simulink model "Rail_PreCtlMeUn"  (R2016b)
settings: configuration reference "CodeGenConfigSet" (kept outside this file)
values from neighbouring files (symbols this model uses):
  Epm_numCyl_C = Calibration.Parameter    [init_Rail_PreCtlMeUn.m]    (also in init_Rail_PreCtlMeUn_SIL.m = Simulink.Parameter)
  PCV_dvolLeak_C = Calibration.Parameter    [init_Rail_PreCtlMeUn.m]    (also in init_Rail_PreCtlMeUn_SIL.m = Simulink.Parameter)
  Rail_dvolLeak_CUR = Calibration.Parameter    [init_Rail_PreCtlMeUn.m]    (also in init_Rail_PreCtlMeUn_SIL.m = Simulink.Parameter)
  Rail_dvolLeak_CURX = Calibration.Parameter    [init_Rail_PreCtlMeUn.m]    (also in init_Rail_PreCtlMeUn_SIL.m = Simulink.Parameter)
  Rail_facDemInjCtlMax_C = Calibration.Parameter    [init_Rail_PreCtlMeUn.m]    (also in init_Rail_PreCtlMeUn_SIL.m = Simulink.Parameter)
  Rail_facLeakEngOn_CUR = Calibration.Parameter    [init_Rail_PreCtlMeUn.m]    (also in init_Rail_PreCtlMeUn_SIL.m = Simulink.Parameter)
  Rail_facLeakEngOn_CURX = Calibration.Parameter    [init_Rail_PreCtlMeUn.m]    (also in init_Rail_PreCtlMeUn_SIL.m = Simulink.Parameter)
  Rail_facLeakTempCor_CUR = Calibration.Parameter    [init_Rail_PreCtlMeUn.m]    (also in init_Rail_PreCtlMeUn_SIL.m = Simulink.Parameter)
  Rail_facLeakTempCor_CURX = Calibration.Parameter    [init_Rail_PreCtlMeUn.m]    (also in init_Rail_PreCtlMeUn_SIL.m = Simulink.Parameter)
  Rail_facPreCtlMeUnCor_MAP = Calibration.Parameter    [init_Rail_PreCtlMeUn.m]    (also in init_Rail_PreCtlMeUn_SIL.m = Simulink.Parameter)
  Rail_facPreCtlMeUnCor_MAPX = Calibration.Parameter    [init_Rail_PreCtlMeUn.m]    (also in init_Rail_PreCtlMeUn_SIL.m = Simulink.Parameter)
  Rail_facPreCtlMeUnCor_MAPY = Calibration.Parameter    [init_Rail_PreCtlMeUn.m]    (also in init_Rail_PreCtlMeUn_SIL.m = Simulink.Parameter)
  Rail_numInjSum_C = Calibration.Parameter    [init_Rail_PreCtlMeUn.m]    (also in init_Rail_PreCtlMeUn_SIL.m = Simulink.Parameter)
  Rail_PreCtlDynKd_C = Calibration.Parameter    [init_Rail_PreCtlMeUn.m]    (also in init_Rail_PreCtlMeUn_SIL.m = Simulink.Parameter)
  Rail_qDemInjCtl_CUR = Calibration.Parameter    [init_Rail_PreCtlMeUn.m]    (also in init_Rail_PreCtlMeUn_SIL.m = Simulink.Parameter)
  Rail_qDemInjCtl_CURX = Calibration.Parameter    [init_Rail_PreCtlMeUn.m]    (also in init_Rail_PreCtlMeUn_SIL.m = Simulink.Parameter)
  Rail_qDemInjCtlMaxOfs_C = Calibration.Parameter    [init_Rail_PreCtlMeUn.m]    (also in init_Rail_PreCtlMeUn_SIL.m = Simulink.Parameter)
  Rail_qPreCtlDynDiffMin_C = Calibration.Parameter    [init_Rail_PreCtlMeUn.m]    (also in init_Rail_PreCtlMeUn_SIL.m = Simulink.Parameter)
  Rail_swtDemInjSel_C = Calibration.Parameter    [init_Rail_PreCtlMeUn.m]    (also in init_Rail_PreCtlMeUn_SIL.m = Simulink.Parameter)
  Rail_tiPreCtlDynT1_C = Calibration.Parameter    [init_Rail_PreCtlMeUn.m]    (also in init_Rail_PreCtlMeUn_SIL.m = Simulink.Parameter)
undefined symbols (not defined in the file or in its folder): EngState_conv, EpmSynState_conv, Rail_PreCtlMeUn_DT
libraries: CXLib x2
settings Model: Creator=lenovo  LastModifiedBy=mayongchao
settings ConfigSetRef: SourceLocation=Base Workspace

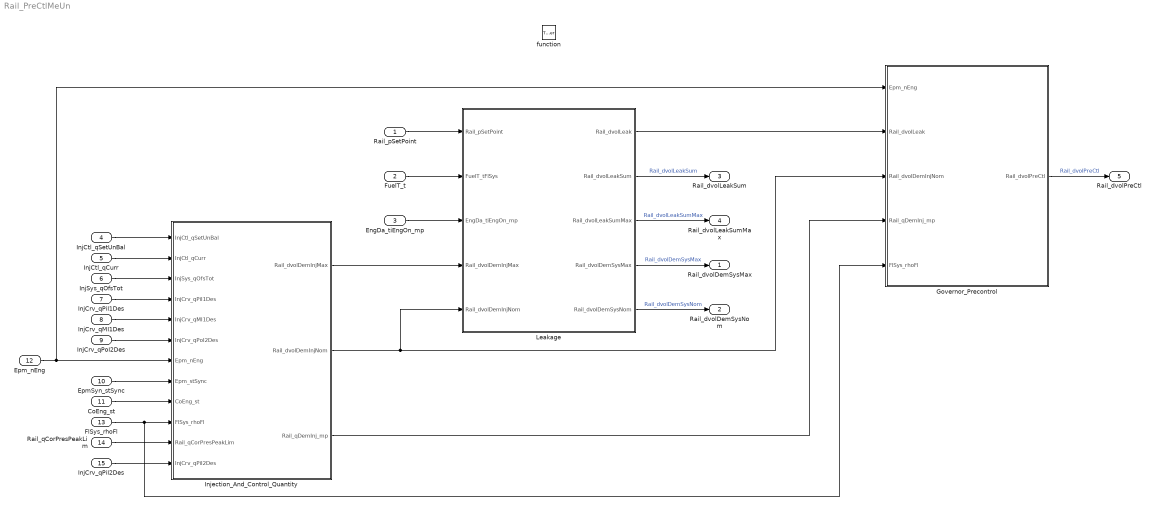
== system Rail_PreCtlMeUn ==
  Rail_pSetPoint : Inport  Tag=bar  Description=Rail pressure setpoint  OutMin=-2500  OutMax=2500  OutDataTypeStr=RailPressure_bar
  FuelT_t : Inport  Tag=deg  Description=Temperature of fuel  Port=2  OutMin=-50  OutMax=150  OutDataTypeStr=Temp_deg
  EngDa_tiEngOn_mp : Inport  Tag=s  Description=Engine on time  Port=3  OutMin=-2147483648  OutMax=2147483647  OutDataTypeStr=TimeEngOn_s
  InjCtl_qSetUnBal : Inport  Tag=mg/hub  Description=Current injection quantity  Port=4  OutMin=-319  OutMax=319  OutDataTypeStr=FuelMass_mg_hub
  InjCtl_qCurr : Inport  Tag=mg/hub  Description=Torque generating engine fuel injection quantity  Port=5  OutMin=-319  OutMax=319  OutDataTypeStr=FuelMass_mg_hub
  InjSys_qOfsTot : Inport  Tag=mg/hub  Description=Non-torque generating quantity, the offset-quantity from torque generating quantity to total quantity  Port=6  OutMin=-319  OutMax=319  OutDataTypeStr=FuelMass_mg_hub
  InjCrv_qPiI1Des : Inport  Tag=mg/hub  Description=Desired PiI injection quantity  Port=7  OutMin=-319  OutMax=319  OutDataTypeStr=FuelMass_mg_hub
  InjCrv_qMI1Des : Inport  Tag=mg/hub  Description=desired MI1 injection quantity  Port=8  OutMin=-319  OutMax=319  OutDataTypeStr=FuelMass_mg_hub
  InjCrv_qPoI2Des : Inport  Tag=mg/hub  Description=Desired PoI2 injection quantity  Port=9  OutMin=-319  OutMax=319  OutDataTypeStr=FuelMass_mg_hub
  EpmSyn_stSync : Inport  Description=state of synchronization  Port=10  OutDataTypeStr=Enum: EpmSynState_conv
  CoEng_st : Inport  Description=Engine coordinator state  Port=11  OutDataTypeStr=Enum: EngState_conv
  Epm_nEng : Inport  Tag=rpm  Description=Engine speed  Port=12  OutMin=0  OutMax=6000  OutDataTypeStr=EngSpeed_rpm
  FlSys_rhoFl : Inport  Tag=kg/m^3  Description=Fuel density coefficient  Port=13  OutMin=0  OutMax=3276  OutDataTypeStr=Fuel_Rho_kg_m3
  Rail_qCorPresPeakLim : Inport  Tag=mg/hub  Description=Quantity correction for limiting pressure peaks (pos. and neg.) mg/cyc  RequirementInfo={'other' 'Rail_requirements.doc' '@Simulink_requirement_item_21' 'true' '（1）根据需求油量选择开关Rail_swtDemInjSel_C选择相应的喷油量作为需求油量。' '' } %GIDa_61847e45_e1c1_4d7b_9351_12b0d31b0ef4  Port=14  OutMin=-300  OutMax=300  OutDataTypeStr=FuelMass_mg_hub
  InjCrv_qPiI2Des : Inport  Tag=mg/hub  Description=Desired PiI injection quantity  RequirementInfo={'other' 'Rail_requirements.doc' '@Simulink_requirement_item_22' 'true' '（2）根据预喷油量和主喷油量查表Rail_qDemInjCtl_CUR，得到相应的控制油量，将两个控制油量相加得到总的控制油量Rail_qDemInjCtlNom_mp。' '' } %GIDa_2488a317_7988_4bfa_9d08_9b42b553773c  Port=15  OutMin=-319  OutMax=319  OutDataTypeStr=FuelMass_mg_hub
  function : TriggerPort  TriggerType=function-call  VariantControl=Variant
  Governor_Precontrol : Subsystem
  Injection_And_Control_Quantity : Subsystem
  Leakage : Subsystem
  Rail_dvolDemSysMax : Outport  Tag=mm^3/s  Description=Volume flow requested overall for a maximum tolerated injection system  OutMin=-327680  OutMax=327670  OutDataTypeStr=FuelVol_mm3_s
  Rail_dvolDemSysNom : Outport  Tag=mm^3/s  Description=Volume flow demanded overall for a nominal injection system  Port=2  OutMin=-327680  OutMax=327670  OutDataTypeStr=FuelVol_mm3_s
  Rail_dvolLeakSum : Outport  Tag=mm^3/s  Description=Summary of Leakages  Port=3  OutMin=-327680  OutMax=327670  OutDataTypeStr=FuelVol_mm3_s
  Rail_dvolLeakSumMax : Outport  Tag=mm^3/s  Description=Lifetime dependant maximum estimated system leakage  Port=4  OutMin=-327680  OutMax=327670  OutDataTypeStr=FuelVol_mm3_s
  Rail_dvolPreCtl : Outport  Tag=mm^3/s  Description=Precontrol value for pressure governing by metering unit  Port=5  OutMin=-327680  OutMax=327670  OutDataTypeStr=FuelVol_mm3_s
  wires:
  Injection_And_Control_Quantity/3(Rail_qDemInj_mp) -> Governor_Precontrol/4(Rail_qDemInj_mp)
  FlSys_rhoFl/1 -> Governor_Precontrol/5(FlSys_rhoFl), Injection_And_Control_Quantity/10(FlSys_rhoFl)
  Governor_Precontrol/1(Rail_dvolPreCtl) -> Rail_dvolPreCtl/1  "Rail_dvolPreCtl"
  Injection_And_Control_Quantity/2(Rail_dvolDemInjNom) -> Leakage/5(Rail_dvolDemInjNom), Governor_Precontrol/3(Rail_dvolDemInjNom)
  Leakage/5(Rail_dvolDemSysNom) -> Rail_dvolDemSysNom/1  "Rail_dvolDemSysNom"
  Leakage/4(Rail_dvolDemSysMax) -> Rail_dvolDemSysMax/1  "Rail_dvolDemSysMax"
  Leakage/3(Rail_dvolLeakSumMax) -> Rail_dvolLeakSumMax/1  "Rail_dvolLeakSumMax"
  Leakage/2(Rail_dvolLeakSum) -> Rail_dvolLeakSum/1  "Rail_dvolLeakSum"
  Leakage/1(Rail_dvolLeak) -> Governor_Precontrol/2(Rail_dvolLeak)
  CoEng_st/1 -> Injection_And_Control_Quantity/9(CoEng_st)
  EpmSyn_stSync/1 -> Injection_And_Control_Quantity/8(Epm_stSync)
  Epm_nEng/1 -> Governor_Precontrol/1(Epm_nEng), Injection_And_Control_Quantity/7(Epm_nEng)
  InjCrv_qMI1Des/1 -> Injection_And_Control_Quantity/5(InjCrv_qMI1Des)
  InjCrv_qPiI1Des/1 -> Injection_And_Control_Quantity/4(InjCrv_qPiI1Des)
  InjSys_qOfsTot/1 -> Injection_And_Control_Quantity/3(InjSys_qOfsTot)
  InjCtl_qSetUnBal/1 -> Injection_And_Control_Quantity/1(InjCtl_qSetUnBal)
  InjCtl_qCurr/1 -> Injection_And_Control_Quantity/2(InjCtl_qCurr)
  FuelT_t/1 -> Leakage/2(FuelT_tFlSys)
  EngDa_tiEngOn_mp/1 -> Leakage/3(EngDa_tiEngOn_mp)
  Rail_pSetPoint/1 -> Leakage/1(Rail_pSetPoint)
  Injection_And_Control_Quantity/1(Rail_dvolDemInjMax) -> Leakage/4(Rail_dvolDemInjMax)
  InjCrv_qPoI2Des/1 -> Injection_And_Control_Quantity/6(InjCrv_qPoI2Des)
  Rail_qCorPresPeakLim/1 -> Injection_And_Control_Quantity/11(Rail_qCorPresPeakLim)
  InjCrv_qPiI2Des/1 -> Injection_And_Control_Quantity/12(InjCrv_qPiI2Des)

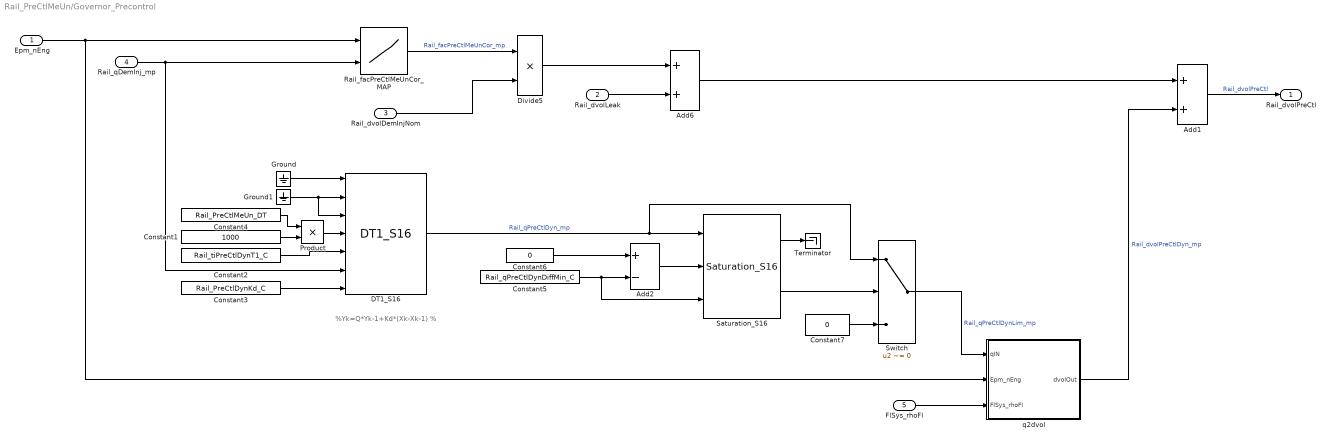
== system Rail_PreCtlMeUn/Governor_Precontrol ==
  note: %Yk=Q*Yk-1+Kd*(Xk-Xk-1) %
  Epm_nEng : Inport  RequirementInfo={'other' 'Rail_requirements.doc' '@Simulink_requirement_item_33' 'true' '基础前馈值' '' } %GIDa_7183900f_2547_4057_a7ba_251e952e1021
  Rail_dvolLeak : Inport  RequirementInfo={'other' 'Rail_requirements.doc' '@Simulink_requirement_item_33' 'true' '基础前馈值' '' } %GIDa_3503d7f1_41ae_4a42_98db_e3eecb9170cb  Port=2
  Rail_dvolDemInjNom : Inport  RequirementInfo={'other' 'Rail_requirements.doc' '@Simulink_requirement_item_33' 'true' '基础前馈值' '' } %GIDa_868a355a_ff47_4d62_936b_22abb35e9b86  Port=3
  Rail_qDemInj_mp : Inport  RequirementInfo={'other' 'Rail_requirements.doc' '@Simulink_requirement_item_33' 'true' '基础前馈值' '' } %GIDa_e1428e79_ed0e_4ba1_a3fd_0a41696d3c11  Port=4
  FlSys_rhoFl : Inport  RequirementInfo={'other' 'Rail_requirements.doc' '@Simulink_requirement_item_34' 'true' '前馈动态补偿体积Rail_dvolPreCtlDyn_mp' '' } %GIDa_798c307b_f932_4494_bf5f_3947ced32dad  Port=5
  Add1 : Sum  InputSameDT=on
  Add2 : Sum  RequirementInfo={'other' 'Rail_requirements.doc' '@Simulink_requirement_item_34' 'true' '前馈动态补偿体积Rail_dvolPreCtlDyn_mp' '' } %GIDa_11a574b0_8317_4258_b280_8d8a7cfa794e  Inputs=+-  InputSameDT=on
  Add6 : Sum  RequirementInfo={'other' 'Rail_requirements.doc' '@Simulink_requirement_item_33' 'true' '基础前馈值' '' } %GIDa_f82aefef_e4ab_49af_af00_2d184f409336  InputSameDT=on
  Constant1 : Constant  RequirementInfo={'other' 'Rail_requirements.doc' '@Simulink_requirement_item_34' 'true' '前馈动态补偿体积Rail_dvolPreCtlDyn_mp' '' } %GIDa_e791a252_ee7e_42c9_85f3_a169ed1ddcc4  Value=1000  OutDataTypeStr=uint16
  Constant2 : Constant  RequirementInfo={'other' 'Rail_requirements.doc' '@Simulink_requirement_item_34' 'true' '前馈动态补偿体积Rail_dvolPreCtlDyn_mp' '' } %GIDa_ec4b6c88_d6b6_478e_9290_0243aa0efb63  Value=Rail_tiPreCtlDynT1_C
  Constant3 : Constant  RequirementInfo={'other' 'Rail_requirements.doc' '@Simulink_requirement_item_34' 'true' '前馈动态补偿体积Rail_dvolPreCtlDyn_mp' '' } %GIDa_c4a7ef06_b727_4a3d_94c2_08782c9b8867  Value=Rail_PreCtlDynKd_C
  Constant4 : Constant  RequirementInfo={'other' 'Rail_requirements.doc' '@Simulink_requirement_item_34' 'true' '前馈动态补偿体积Rail_dvolPreCtlDyn_mp' '' } %GIDa_1b5483ab_5d1d_41df_9217_4aee7852aaf8  Value=Rail_PreCtlMeUn_DT  OutDataTypeStr=uint16
  Constant5 : Constant  RequirementInfo={'other' 'Rail_requirements.doc' '@Simulink_requirement_item_34' 'true' '前馈动态补偿体积Rail_dvolPreCtlDyn_mp' '' } %GIDa_54dd0a63_7d23_407e_aac7_70a39433bdd0  Value=Rail_qPreCtlDynDiffMin_C
  Constant6 : Constant  RequirementInfo={'other' 'Rail_requirements.doc' '@Simulink_requirement_item_34' 'true' '前馈动态补偿体积Rail_dvolPreCtlDyn_mp' '' } %GIDa_20ac7aa5_ee3b_45c0_9ed5_4f6856be27d3  Value=0  OutDataTypeStr=Inherit: Inherit via back propagation
  Constant7 : Constant  RequirementInfo={'other' 'Rail_requirements.doc' '@Simulink_requirement_item_34' 'true' '前馈动态补偿体积Rail_dvolPreCtlDyn_mp' '' } %GIDa_dbe14c56_3d27_499d_a0c9_6c8275566cb4  Value=0  OutDataTypeStr=Inherit: Inherit via back propagation
  DT1_S16 : CXLib/DT1_S16  RequirementInfo={'other' 'Rail_requirements.doc' '@Simulink_requirement_item_34' 'true' '前馈动态补偿体积Rail_dvolPreCtlDyn_mp' '' } %GIDa_61af2057_1ae7_4294_9d8b_88d75294bae1
  Divide5 : Product  RequirementInfo={'other' 'Rail_requirements.doc' '@Simulink_requirement_item_33' 'true' '基础前馈值' '' } %GIDa_4ce6a312_6fe6_46db_860a_63764939d657  Inputs=**  OutDataTypeStr=FuelVol_mm3_s
  Ground : Ground  RequirementInfo={'other' 'Rail_requirements.doc' '@Simulink_requirement_item_34' 'true' '前馈动态补偿体积Rail_dvolPreCtlDyn_mp' '' } %GIDa_0a4a3791_a005_4ed8_981b_586e8985940b
  Ground1 : Ground  RequirementInfo={'other' 'Rail_requirements.doc' '@Simulink_requirement_item_34' 'true' '前馈动态补偿体积Rail_dvolPreCtlDyn_mp' '' } %GIDa_2de3f24a_c7b3_45e3_9504_81736252fde4
  Product : Product  OutDataTypeStr=uint32
  Rail_facPreCtlMeUnCor_MAP : Lookup_n-D  RequirementInfo={'other' 'Rail_requirements.doc' '@Simulink_requirement_item_33' 'true' '基础前馈值' '' } %GIDa_8b072701_d5e1_45ce_8885_5bebdd0f4c2d  BreakpointsForDimension1=Rail_facPreCtlMeUnCor_MAPY  BreakpointsForDimension2=Rail_facPreCtlMeUnCor_MAPX  IndexSearchMethod=Linear search  Table=Rail_facPreCtlMeUnCor_MAP  ExtrapMethod=Clip  InternalRulePriority=Speed  OutDataTypeStr=Inherit: Inherit via back propagation  RndMeth=Simplest  SaturateOnIntegerOverflow=on
  Saturation_S16 : CXLib/Saturation_S16  RequirementInfo={'other' 'Rail_requirements.doc' '@Simulink_requirement_item_34' 'true' '前馈动态补偿体积Rail_dvolPreCtlDyn_mp' '' } %GIDa_899e831a_b92b_45e4_b5c0_482f008df581
  Switch : Switch  Criteria=u2 ~= 0  OutDataTypeStr=Inherit: Inherit via back propagation
  Terminator : Terminator
  q2dvol : Subsystem
  Rail_dvolPreCtl : Outport
  wires:
  DT1_S16/1 -> Switch/1, Saturation_S16/1  "Rail_qPreCtlDyn_mp"
  Constant3/1 -> DT1_S16/7
  Constant2/1 -> DT1_S16/5
  FlSys_rhoFl/1 -> q2dvol/3(FlSys_rhoFl)
  Add1/1 -> Rail_dvolPreCtl/1  "Rail_dvolPreCtl"
  q2dvol/1(dvolOut) -> Add1/2  "Rail_dvolPreCtlDyn_mp"
  Add2/1 -> Saturation_S16/2
  Constant6/1 -> Add2/1
  Constant5/1 -> Saturation_S16/3, Add2/2
  Ground1/1 -> DT1_S16/3, DT1_S16/2
  Ground/1 -> DT1_S16/1
  Add6/1 -> Add1/1
  Rail_dvolLeak/1 -> Add6/2
  Divide5/1 -> Add6/1
  Rail_dvolDemInjNom/1 -> Divide5/2
  Rail_facPreCtlMeUnCor_MAP/1 -> Divide5/1  "Rail_facPreCtlMeUnCor_mp"
  Rail_qDemInj_mp/1 -> Rail_facPreCtlMeUnCor_MAP/2, DT1_S16/6
  Epm_nEng/1 -> q2dvol/2(Epm_nEng), Rail_facPreCtlMeUnCor_MAP/1
  Product/1 -> DT1_S16/4
  Constant1/1 -> Product/2
  Constant4/1 -> Product/1
  Switch/1 -> q2dvol/1(qIN)  "Rail_qPreCtlDynLim_mp"
  Saturation_S16/2 -> Switch/2
  Saturation_S16/1 -> Terminator/1
  Constant7/1 -> Switch/3

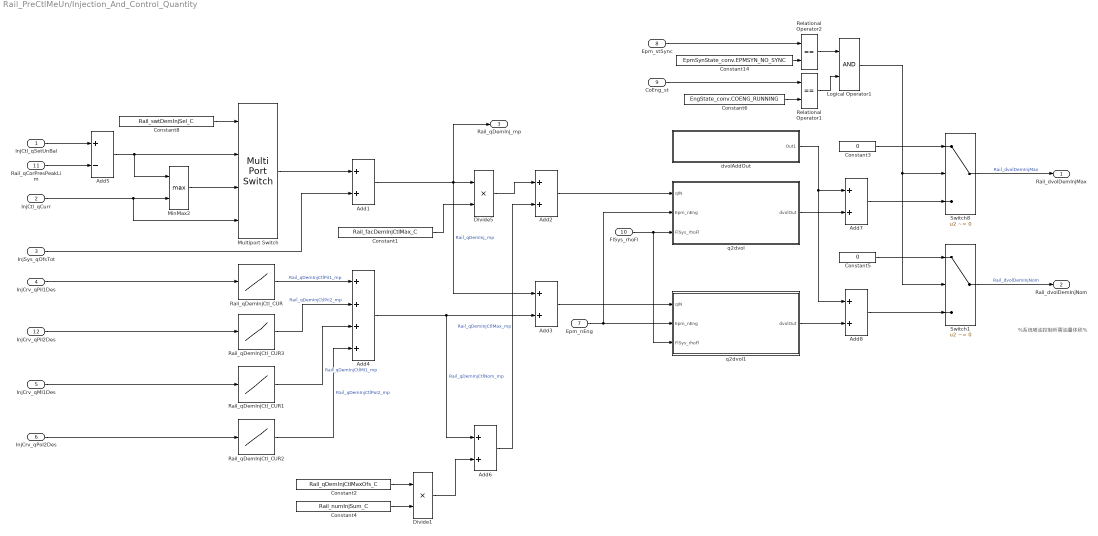
== system Rail_PreCtlMeUn/Injection_And_Control_Quantity ==
  note: %系统喷油控制所需油量体积%
  InjCtl_qSetUnBal : Inport  RequirementInfo={'other' 'Rail_requirements.doc' '@Simulink_requirement_item_21' 'true' '（1）根据需求油量选择开关Rail_swtDemInjSel_C选择相应的喷油量作为需求油量。' '' } %GIDa_d86a20ce_fc14_4f42_8307_85335138969d
  InjCtl_qCurr : Inport  RequirementInfo={'other' 'Rail_requirements.doc' '@Simulink_requirement_item_21' 'true' '（1）根据需求油量选择开关Rail_swtDemInjSel_C选择相应的喷油量作为需求油量。' '' } %GIDa_70742e20_ac76_4111_a9ad_54025b245dd1  Port=2
  InjSys_qOfsTot : Inport  RequirementInfo={'other' 'Rail_requirements.doc' '@Simulink_requirement_item_21' 'true' '（1）根据需求油量选择开关Rail_swtDemInjSel_C选择相应的喷油量作为需求油量。' '' } %GIDa_0d9af8d7_e83d_46c0_829a_4f6a44006e6d  Port=3
  InjCrv_qPiI1Des : Inport  RequirementInfo={'other' 'Rail_requirements.doc' '@Simulink_requirement_item_22' 'true' '（2）根据预喷油量和主喷油量查表Rail_qDemInjCtl_CUR，得到相应的控制油量，将两个控制油量相加得到总的控制油量Rail_qDemInjCtlNom_mp。' '' } %GIDa_605ee073_d6d5_4205_a4e2_e10b92a8f3d8  Port=4
  InjCrv_qMI1Des : Inport  RequirementInfo={'other' 'Rail_requirements.doc' '@Simulink_requirement_item_22' 'true' '（2）根据预喷油量和主喷油量查表Rail_qDemInjCtl_CUR，得到相应的控制油量，将两个控制油量相加得到总的控制油量Rail_qDemInjCtlNom_mp。' '' } %GIDa_c13542f0_9b00_48f8_9292_7fb6c80c9909  Port=5
  InjCrv_qPoI2Des : Inport  RequirementInfo={'other' 'Rail_requirements.doc' '@Simulink_requirement_item_22' 'true' '（2）根据预喷油量和主喷油量查表Rail_qDemInjCtl_CUR，得到相应的控制油量，将两个控制油量相加得到总的控制油量Rail_qDemInjCtlNom_mp。' '' } %GIDa_8e2944c1_08cb_41db_9afa_bc38b111ab4f  Port=6
  Epm_nEng : Inport  Port=7
  Epm_stSync : Inport  RequirementInfo={'other' 'Rail_requirements.doc' '@Simulink_requirement_item_25' 'true' '（5）当发动机正常运行，而ECU处于非同步状态时，系统总需求油量体积和最大进油体积均设为0。' '' } %GIDa_7bbab8b7_1d9f_4eeb_98b8_6fc4d458bffa  Port=8
  CoEng_st : Inport  RequirementInfo={'other' 'Rail_requirements.doc' '@Simulink_requirement_item_25' 'true' '（5）当发动机正常运行，而ECU处于非同步状态时，系统总需求油量体积和最大进油体积均设为0。' '' } %GIDa_02f05315_acfb_40b1_98c7_9dfcad1dc704  Port=9
  FlSys_rhoFl : Inport  Port=10
  Rail_qCorPresPeakLim : Inport  RequirementInfo={'other' 'Rail_requirements.doc' '@Simulink_requirement_item_21' 'true' '（1）根据需求油量选择开关Rail_swtDemInjSel_C选择相应的喷油量作为需求油量。' '' } %GIDa_170ec101_d649_4438_832f_5aabf0feb4fb  Port=11
  InjCrv_qPiI2Des : Inport  RequirementInfo={'other' 'Rail_requirements.doc' '@Simulink_requirement_item_22' 'true' '（2）根据预喷油量和主喷油量查表Rail_qDemInjCtl_CUR，得到相应的控制油量，将两个控制油量相加得到总的控制油量Rail_qDemInjCtlNom_mp。' '' } %GIDa_965be6ba_45da_4819_acd6_c12ba0b01220  Port=12
  Add1 : Sum  RequirementInfo={'other' 'Rail_requirements.doc' '@Simulink_requirement_item_21' 'true' '（1）根据需求油量选择开关Rail_swtDemInjSel_C选择相应的喷油量作为需求油量。' '' } %GIDa_f4dbabbe_6e8f_4f94_a6be_f7a604a8bd49  InputSameDT=on
  Add2 : Sum  InputSameDT=on
  Add3 : Sum  InputSameDT=on
  Add4 : Sum  RequirementInfo={'other' 'Rail_requirements.doc' '@Simulink_requirement_item_22' 'true' '（2）根据预喷油量和主喷油量查表Rail_qDemInjCtl_CUR，得到相应的控制油量，将两个控制油量相加得到总的控制油量Rail_qDemInjCtlNom_mp。' '' } %GIDa_adfa47f0_97ff_44db_9dac_65136f99c460  Inputs=++++  InputSameDT=on
  Add5 : Sum  RequirementInfo={'other' 'Rail_requirements.doc' '@Simulink_requirement_item_21' 'true' '（1）根据需求油量选择开关Rail_swtDemInjSel_C选择相应的喷油量作为需求油量。' '' } %GIDa_65a978d3_fbe9_4f76_ab00_448c534e4306  Inputs=+-  OutDataTypeStr=Inherit: Inherit via back propagation  InputSameDT=on
  Add6 : Sum  RequirementInfo={'other' 'Rail_requirements.doc' '@Simulink_requirement_item_23' 'true' '（3）为适应系统老化，需预估一个最大控制油量Rail_qDemInjCtlMax_mp，从而保护燃油计量阀和高压油泵。' '' } %GIDa_e21f69a2_9c3e_4ad7_9a9c_34ddffd467c8  InputSameDT=on
  Add7 : Sum  OutDataTypeStr=Inherit: Inherit via back propagation  InputSameDT=on
  Add8 : Sum  OutDataTypeStr=Inherit: Inherit via back propagation  InputSameDT=on
  Constant1 : Constant  RequirementInfo={'other' 'Rail_requirements.doc' '@Simulink_requirement_item_23' 'true' '（3）为适应系统老化，需预估一个最大控制油量Rail_qDemInjCtlMax_mp，从而保护燃油计量阀和高压油泵。' '' } %GIDa_bbcf7b1e_4515_4b0c_bebc_f19409aea922  Value=Rail_facDemInjCtlMax_C
  Constant14 : Constant  RequirementInfo={'other' 'Rail_requirements.doc' '@Simulink_requirement_item_25' 'true' '（5）当发动机正常运行，而ECU处于非同步状态时，系统总需求油量体积和最大进油体积均设为0。' '' } %GIDa_9552abac_9906_4052_a970_80518a916d99  Value=EpmSynState_conv.EPMSYN_NO_SYNC
  Constant2 : Constant  RequirementInfo={'other' 'Rail_requirements.doc' '@Simulink_requirement_item_23' 'true' '（3）为适应系统老化，需预估一个最大控制油量Rail_qDemInjCtlMax_mp，从而保护燃油计量阀和高压油泵。' '' } %GIDa_daf2c207_8c8f_404c_9cb7_f3f854fab4c5  Value=Rail_qDemInjCtlMaxOfs_C
  Constant3 : Constant  RequirementInfo={'other' 'Rail_requirements.doc' '@Simulink_requirement_item_25' 'true' '（5）当发动机正常运行，而ECU处于非同步状态时，系统总需求油量体积和最大进油体积均设为0。' '' } %GIDa_96f668b4_60b5_4517_a7ce_91f2089a44c7  Value=0  OutDataTypeStr=Inherit: Inherit via back propagation
  Constant4 : Constant  RequirementInfo={'other' 'Rail_requirements.doc' '@Simulink_requirement_item_23' 'true' '（3）为适应系统老化，需预估一个最大控制油量Rail_qDemInjCtlMax_mp，从而保护燃油计量阀和高压油泵。' '' } %GIDa_4479e7d4_2469_4e06_9e03_04d5cb1c27b3  Value=Rail_numInjSum_C
  Constant5 : Constant  RequirementInfo={'other' 'Rail_requirements.doc' '@Simulink_requirement_item_25' 'true' '（5）当发动机正常运行，而ECU处于非同步状态时，系统总需求油量体积和最大进油体积均设为0。' '' } %GIDa_b23e15b2_8a91_45f4_9403_a6bac7d964f9  Value=0  OutDataTypeStr=Inherit: Inherit via back propagation
  Constant6 : Constant  RequirementInfo={'other' 'Rail_requirements.doc' '@Simulink_requirement_item_25' 'true' '（5）当发动机正常运行，而ECU处于非同步状态时，系统总需求油量体积和最大进油体积均设为0。' '' } %GIDa_a94b91ee_a0ec_4101_a821_07718b3495e9  Value=EngState_conv.COENG_RUNNING
  Constant8 : Constant  RequirementInfo={'other' 'Rail_requirements.doc' '@Simulink_requirement_item_21' 'true' '（1）根据需求油量选择开关Rail_swtDemInjSel_C选择相应的喷油量作为需求油量。' '' } %GIDa_d575464b_40e6_44a7_91f7_7bf9b62d767f  Value=Rail_swtDemInjSel_C
  Divide1 : Product  RequirementInfo={'other' 'Rail_requirements.doc' '@Simulink_requirement_item_23' 'true' '（3）为适应系统老化，需预估一个最大控制油量Rail_qDemInjCtlMax_mp，从而保护燃油计量阀和高压油泵。' '' } %GIDa_51dcb6dc_d348_474e_8a9b_c3373ee273d7  Inputs=**  OutDataTypeStr=FuelMass_mg_hub
  Divide5 : Product  RequirementInfo={'other' 'Rail_requirements.doc' '@Simulink_requirement_item_23' 'true' '（3）为适应系统老化，需预估一个最大控制油量Rail_qDemInjCtlMax_mp，从而保护燃油计量阀和高压油泵。' '' } %GIDa_5a2e9475_bd3a_4967_81da_71b5b144bfc3  Inputs=**  OutDataTypeStr=FuelMass_mg_hub
  Logical Operator1 : Logic  RequirementInfo={'other' 'Rail_requirements.doc' '@Simulink_requirement_item_25' 'true' '（5）当发动机正常运行，而ECU处于非同步状态时，系统总需求油量体积和最大进油体积均设为0。' '' } %GIDa_4659d2aa_f293_4665_bbd0_3b36f4efba34  AllPortsSameDT=off  OutDataTypeStr=boolean
  MinMax2 : MinMax  RequirementInfo={'other' 'Rail_requirements.doc' '@Simulink_requirement_item_21' 'true' '（1）根据需求油量选择开关Rail_swtDemInjSel_C选择相应的喷油量作为需求油量。' '' } %GIDa_9ebeef09_b96f_45e9_b405_950b078767d4  Function=max  Inputs=2  InputSameDT=on
  Multiport Switch : MultiPortSwitch  RequirementInfo={'other' 'Rail_requirements.doc' '@Simulink_requirement_item_21' 'true' '（1）根据需求油量选择开关Rail_swtDemInjSel_C选择相应的喷油量作为需求油量。' '' } %GIDa_68e80737_64ed_4998_bda0_42d24ba91242  DiagnosticForDefault=None  InputSameDT=on
  Rail_qDemInjCtl_CUR : Lookup_n-D  RequirementInfo={'other' 'Rail_requirements.doc' '@Simulink_requirement_item_22' 'true' '（2）根据预喷油量和主喷油量查表Rail_qDemInjCtl_CUR，得到相应的控制油量，将两个控制油量相加得到总的控制油量Rail_qDemInjCtlNom_mp。' '' } %GIDa_c473b0e9_2d7e_4972_a936_f7983c5b344c  NumberOfTableDimensions=1  BreakpointsForDimension1=Rail_qDemInjCtl_CURX  IndexSearchMethod=Linear search  Table=Rail_qDemInjCtl_CUR  ExtrapMethod=Clip  InternalRulePriority=Speed  OutDataTypeStr=Inherit: Inherit via back propagation  RndMeth=Simplest  SaturateOnIntegerOverflow=on
  Rail_qDemInjCtl_CUR1 : Lookup_n-D  RequirementInfo={'other' 'Rail_requirements.doc' '@Simulink_requirement_item_22' 'true' '（2）根据预喷油量和主喷油量查表Rail_qDemInjCtl_CUR，得到相应的控制油量，将两个控制油量相加得到总的控制油量Rail_qDemInjCtlNom_mp。' '' } %GIDa_acdf9868_7481_41f7_b158_cb4908adafe2  NumberOfTableDimensions=1  BreakpointsForDimension1=Rail_qDemInjCtl_CURX  IndexSearchMethod=Linear search  Table=Rail_qDemInjCtl_CUR  ExtrapMethod=Clip  InternalRulePriority=Speed  OutDataTypeStr=Inherit: Inherit via back propagation  RndMeth=Simplest  SaturateOnIntegerOverflow=on
  Rail_qDemInjCtl_CUR2 : Lookup_n-D  RequirementInfo={'other' 'Rail_requirements.doc' '@Simulink_requirement_item_22' 'true' '（2）根据预喷油量和主喷油量查表Rail_qDemInjCtl_CUR，得到相应的控制油量，将两个控制油量相加得到总的控制油量Rail_qDemInjCtlNom_mp。' '' } %GIDa_3f07b9d5_860a_440b_aab4_5710e3e3b534  NumberOfTableDimensions=1  BreakpointsForDimension1=Rail_qDemInjCtl_CURX  IndexSearchMethod=Linear search  Table=Rail_qDemInjCtl_CUR  ExtrapMethod=Clip  InternalRulePriority=Speed  OutDataTypeStr=Inherit: Inherit via back propagation  RndMeth=Simplest  SaturateOnIntegerOverflow=on
  Rail_qDemInjCtl_CUR3 : Lookup_n-D  RequirementInfo={'other' 'Rail_requirements.doc' '@Simulink_requirement_item_22' 'true' '（2）根据预喷油量和主喷油量查表Rail_qDemInjCtl_CUR，得到相应的控制油量，将两个控制油量相加得到总的控制油量Rail_qDemInjCtlNom_mp。' '' } %GIDa_fc070bfc_f840_4fa2_9623_31a7235dfc74  NumberOfTableDimensions=1  BreakpointsForDimension1=Rail_qDemInjCtl_CURX  IndexSearchMethod=Linear search  Table=Rail_qDemInjCtl_CUR  ExtrapMethod=Clip  InternalRulePriority=Speed  OutDataTypeStr=Inherit: Inherit via back propagation  RndMeth=Simplest  SaturateOnIntegerOverflow=on
  Relational Operator1 : RelationalOperator  RequirementInfo={'other' 'Rail_requirements.doc' '@Simulink_requirement_item_25' 'true' '（5）当发动机正常运行，而ECU处于非同步状态时，系统总需求油量体积和最大进油体积均设为0。' '' } %GIDa_e77ae7fd_c40f_489e_88b8_3d506b56b9f9  Operator===  OutDataTypeStr=boolean  RndMeth=Nearest  InputSameDT=on
  Relational Operator2 : RelationalOperator  RequirementInfo={'other' 'Rail_requirements.doc' '@Simulink_requirement_item_25' 'true' '（5）当发动机正常运行，而ECU处于非同步状态时，系统总需求油量体积和最大进油体积均设为0。' '' } %GIDa_97c7a11d_d6ce_491a_b19a_2d9af0a8132d  Operator===  OutDataTypeStr=boolean  RndMeth=Nearest  InputSameDT=on
  Switch1 : Switch  RequirementInfo={'other' 'Rail_requirements.doc' '@Simulink_requirement_item_25' 'true' '（5）当发动机正常运行，而ECU处于非同步状态时，系统总需求油量体积和最大进油体积均设为0。' '' } %GIDa_dca91527_9475_4f6b_9738_6077bd162fe9  Criteria=u2 ~= 0  InputSameDT=on
  Switch8 : Switch  RequirementInfo={'other' 'Rail_requirements.doc' '@Simulink_requirement_item_25' 'true' '（5）当发动机正常运行，而ECU处于非同步状态时，系统总需求油量体积和最大进油体积均设为0。' '' } %GIDa_2182196c_e831_4db3_9b6a_a227ccbc258e  Criteria=u2 ~= 0  InputSameDT=on
  dvolAddOut : Subsystem  RequirementInfo={'other' 'Rail_requirements.doc' '@Simulink_requirement_item_24' 'true' '（4）为了得到相应的需求油量体积，需将油量经过q2dvol模块转换成体积单位。' '' } %GIDa_55f88d7a_6274_4a51_a261_5d02fc687ec0
  q2dvol : Subsystem
  q2dvol1 : Subsystem
  Rail_dvolDemInjMax : Outport  RequirementInfo={'other' 'Rail_requirements.doc' '@Simulink_requirement_item_25' 'true' '（5）当发动机正常运行，而ECU处于非同步状态时，系统总需求油量体积和最大进油体积均设为0。' '' } %GIDa_69e3ef99_5850_4012_bc80_fd8ca58c444c
  Rail_dvolDemInjNom : Outport  RequirementInfo={'other' 'Rail_requirements.doc' '@Simulink_requirement_item_25' 'true' '（5）当发动机正常运行，而ECU处于非同步状态时，系统总需求油量体积和最大进油体积均设为0。' '' } %GIDa_832e3d6e_97e1_4663_ae38_4900a203a95e  Port=2
  Rail_qDemInj_mp : Outport  Port=3
  wires:
  Add2/1 -> q2dvol/1(qIN)
  FlSys_rhoFl/1 -> q2dvol1/3(FlSys_rhoFl), q2dvol/3(FlSys_rhoFl)
  Constant8/1 -> Multiport Switch/1
  Logical Operator1/1 -> Switch8/2, Switch1/2
  CoEng_st/1 -> Relational Operator1/1
  Constant6/1 -> Relational Operator1/2
  Relational Operator1/1 -> Logical Operator1/2
  Epm_stSync/1 -> Relational Operator2/1
  Constant14/1 -> Relational Operator2/2
  Relational Operator2/1 -> Logical Operator1/1
  Switch1/1 -> Rail_dvolDemInjNom/1  "Rail_dvolDemInjNom"
  Constant5/1 -> Switch1/1
  Add8/1 -> Switch1/3
  Switch8/1 -> Rail_dvolDemInjMax/1  "Rail_dvolDemInjMax"
  Constant3/1 -> Switch8/1
  Add7/1 -> Switch8/3
  dvolAddOut/1(Out1) -> Add7/1, Add8/1
  q2dvol1/1(dvolOut) -> Add8/2
  q2dvol/1(dvolOut) -> Add7/2
  Epm_nEng/1 -> q2dvol1/2(Epm_nEng), q2dvol/2(Epm_nEng)
  Add3/1 -> q2dvol1/1(qIN)
  Add6/1 -> Add2/2  "Rail_qDemInjCtlMax_mp"
  Divide1/1 -> Add6/2
  Constant2/1 -> Divide1/1
  Constant1/1 -> Divide5/2
  Add4/1 -> Add6/1, Add3/2  "Rail_qDemInjCtlNom_mp"
  Rail_qDemInjCtl_CUR1/1 -> Add4/3  "Rail_qDemInjCtlMI1_mp"
  Rail_qDemInjCtl_CUR/1 -> Add4/1  "Rail_qDemInjCtlPiI1_mp"
  InjCrv_qMI1Des/1 -> Rail_qDemInjCtl_CUR1/1
  InjCrv_qPiI1Des/1 -> Rail_qDemInjCtl_CUR/1
  Add1/1 -> Divide5/1, Rail_qDemInj_mp/1, Add3/1  "Rail_qDemInj_mp"
  Multiport Switch/1 -> Add1/1
  InjSys_qOfsTot/1 -> Add1/2
  InjCtl_qCurr/1 -> MinMax2/2, Multiport Switch/4
  MinMax2/1 -> Multiport Switch/3
  Add5/1 -> Multiport Switch/2, MinMax2/1
  InjCtl_qSetUnBal/1 -> Add5/1
  Rail_qCorPresPeakLim/1 -> Add5/2
  Constant4/1 -> Divide1/2
  InjCrv_qPoI2Des/1 -> Rail_qDemInjCtl_CUR2/1
  Rail_qDemInjCtl_CUR2/1 -> Add4/4  "Rail_qDemInjCtlPoI2_mp"
  Divide5/1 -> Add2/1
  Rail_qDemInjCtl_CUR3/1 -> Add4/2  "Rail_qDemInjCtlPiI2_mp"
  InjCrv_qPiI2Des/1 -> Rail_qDemInjCtl_CUR3/1

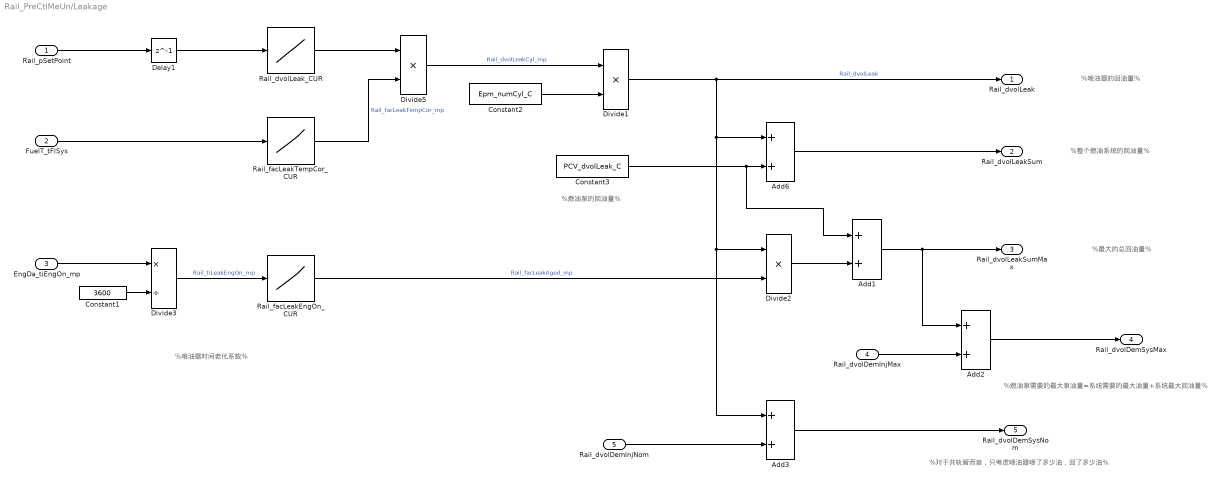
== system Rail_PreCtlMeUn/Leakage ==
  note: %喷油器时间老化系数%
  note: %喷油器的回油量%
  note: %燃油泵的回油量%
  note: %最大的总回油量%
  note: %燃油泵需要的最大泵油量=系统需要的最大油量+系统最大回油量%
  note: %整个燃油系统的回油量%
  note: %对于共轨管而言，只考虑喷油器喷了多少油，回了多少油%
  Rail_pSetPoint : Inport  RequirementInfo={'other' 'Rail_requirements.doc' '@Simulink_requirement_item_27' 'true' '喷油器总共的回油量Rail_dvolLeak' '' } %GIDa_405693ea_d255_4b01_b311_18e27d2ea0d1
  FuelT_tFlSys : Inport  RequirementInfo={'other' 'Rail_requirements.doc' '@Simulink_requirement_item_27' 'true' '喷油器总共的回油量Rail_dvolLeak' '' } %GIDa_6f18efd1_0955_4838_b382_633712ab90fb  Port=2
  EngDa_tiEngOn_mp : Inport  RequirementInfo={'other' 'Rail_requirements.doc' '@Simulink_requirement_item_29' 'true' '系统最大回油量Rail_dvolLeakSumMax' '' } %GIDa_68a86d51_4f04_419b_a5e0_2dc97734195a  Port=3
  Rail_dvolDemInjMax : Inport  RequirementInfo={'other' 'Rail_requirements.doc' '@Simulink_requirement_item_30' 'true' '燃油泵需要的最大泵油体积Rail_dvolDemSysMax' '' } %GIDa_8dbeca4d_bb56_48a4_96cb_db3b3bc8e360  Port=4
  Rail_dvolDemInjNom : Inport  RequirementInfo={'other' 'Rail_requirements.doc' '@Simulink_requirement_item_31' 'true' '系统正常工况下需要的泵油体积Rail_dvolDemSysNom' '' } %GIDa_ed262064_8bf1_46cb_bd6f_c0615dbbaf4e  Port=5
  Add1 : Sum  RequirementInfo={'other' 'Rail_requirements.doc' '@Simulink_requirement_item_29' 'true' '系统最大回油量Rail_dvolLeakSumMax' '' } %GIDa_a3d6e970_65dc_4038_b356_82c6d6bd33fb  InputSameDT=on
  Add2 : Sum  RequirementInfo={'other' 'Rail_requirements.doc' '@Simulink_requirement_item_30' 'true' '燃油泵需要的最大泵油体积Rail_dvolDemSysMax' '' } %GIDa_a4fae57f_0058_4b68_822d_7556306547a0  InputSameDT=on
  Add3 : Sum  RequirementInfo={'other' 'Rail_requirements.doc' '@Simulink_requirement_item_31' 'true' '系统正常工况下需要的泵油体积Rail_dvolDemSysNom' '' } %GIDa_6f42a25b_1e90_48bd_8b73_b1418cc90d3c  InputSameDT=on
  Add6 : Sum  RequirementInfo={'other' 'Rail_requirements.doc' '@Simulink_requirement_item_28' 'true' '系统总的回油量Rail_dvolLeakSum' '' } %GIDa_dcc1c622_d94c_4993_be4a_374f224e360e  InputSameDT=on
  Constant1 : Constant  RequirementInfo={'other' 'Rail_requirements.doc' '@Simulink_requirement_item_29' 'true' '系统最大回油量Rail_dvolLeakSumMax' '' } %GIDa_25c008e4_23d2_4fa8_b169_daea8c2fa189  Value=3600  OutDataTypeStr=Inherit: Inherit via back propagation
  Constant2 : Constant  Value=Epm_numCyl_C
  Constant3 : Constant  Value=PCV_dvolLeak_C
  Delay1 : Delay  DelayLength=1  InitialCondition=0
  Divide1 : Product  RequirementInfo={'other' 'Rail_requirements.doc' '@Simulink_requirement_item_27' 'true' '喷油器总共的回油量Rail_dvolLeak' '' } %GIDa_90cb2014_38bf_451d_b816_c52a755bd4cc  Inputs=**  OutDataTypeStr=FuelVol_mm3_s
  Divide2 : Product  RequirementInfo={'other' 'Rail_requirements.doc' '@Simulink_requirement_item_29' 'true' '系统最大回油量Rail_dvolLeakSumMax' '' } %GIDa_38381203_eb71_4945_bc5b_3f8fb5b5a7bc  Inputs=**  OutDataTypeStr=FuelVol_mm3_s
  Divide3 : Product  RequirementInfo={'other' 'Rail_requirements.doc' '@Simulink_requirement_item_29' 'true' '系统最大回油量Rail_dvolLeakSumMax' '' } %GIDa_cdd53ebd_4542_4f65_8467_fe001fe80a12  Inputs=*/  OutDataTypeStr=RailHrsEngOn_h
  Divide5 : Product  RequirementInfo={'other' 'Rail_requirements.doc' '@Simulink_requirement_item_27' 'true' '喷油器总共的回油量Rail_dvolLeak' '' } %GIDa_a4e6ea36_1026_4e07_ae2d_ccab7b9dde0d  Inputs=**  OutDataTypeStr=FuelVol_mm3_s
  Rail_dvolLeak_CUR : Lookup_n-D  RequirementInfo={'other' 'Rail_requirements.doc' '@Simulink_requirement_item_27' 'true' '喷油器总共的回油量Rail_dvolLeak' '' } %GIDa_3fd3d2ec_340a_4253_8f58_36cdb97a7230  NumberOfTableDimensions=1  BreakpointsForDimension1=Rail_dvolLeak_CURX  IndexSearchMethod=Linear search  Table=Rail_dvolLeak_CUR  ExtrapMethod=Clip  InternalRulePriority=Speed  OutDataTypeStr=Inherit: Inherit via back propagation  RndMeth=Simplest  SaturateOnIntegerOverflow=on
  Rail_facLeakEngOn_CUR : Lookup_n-D  RequirementInfo={'other' 'Rail_requirements.doc' '@Simulink_requirement_item_29' 'true' '系统最大回油量Rail_dvolLeakSumMax' '' } %GIDa_425b614b_ec52_4206_95ad_cec9e809cdc2  NumberOfTableDimensions=1  BreakpointsForDimension1=Rail_facLeakEngOn_CURX  IndexSearchMethod=Linear search  Table=Rail_facLeakEngOn_CUR  ExtrapMethod=Clip  InternalRulePriority=Speed  OutDataTypeStr=Inherit: Inherit via back propagation  RndMeth=Simplest  SaturateOnIntegerOverflow=on
  Rail_facLeakTempCor_CUR : Lookup_n-D  RequirementInfo={'other' 'Rail_requirements.doc' '@Simulink_requirement_item_27' 'true' '喷油器总共的回油量Rail_dvolLeak' '' } %GIDa_cc2428ed_cc17_4906_a451_78bc980306a5  NumberOfTableDimensions=1  BreakpointsForDimension1=Rail_facLeakTempCor_CURX  IndexSearchMethod=Linear search  Table=Rail_facLeakTempCor_CUR  ExtrapMethod=Clip  InternalRulePriority=Speed  OutDataTypeStr=Inherit: Inherit via back propagation  RndMeth=Simplest  SaturateOnIntegerOverflow=on
  Rail_dvolLeak : Outport  RequirementInfo={'other' 'Rail_requirements.doc' '@Simulink_requirement_item_27' 'true' '喷油器总共的回油量Rail_dvolLeak' '' } %GIDa_37ace723_0103_49d4_a4d8_db5a6f49ce8c
  Rail_dvolLeakSum : Outport  RequirementInfo={'other' 'Rail_requirements.doc' '@Simulink_requirement_item_28' 'true' '系统总的回油量Rail_dvolLeakSum' '' } %GIDa_cd965c42_0937_48ea_a056_6031247f1efa  Port=2
  Rail_dvolLeakSumMax : Outport  RequirementInfo={'other' 'Rail_requirements.doc' '@Simulink_requirement_item_29' 'true' '系统最大回油量Rail_dvolLeakSumMax' '' } %GIDa_72429436_6d39_4f49_af2c_1c980fd55f5b  Port=3
  Rail_dvolDemSysMax : Outport  RequirementInfo={'other' 'Rail_requirements.doc' '@Simulink_requirement_item_30' 'true' '燃油泵需要的最大泵油体积Rail_dvolDemSysMax' '' } %GIDa_17bff9d7_2d7e_4da4_be11_297f19622f5a  Port=4
  Rail_dvolDemSysNom : Outport  RequirementInfo={'other' 'Rail_requirements.doc' '@Simulink_requirement_item_31' 'true' '系统正常工况下需要的泵油体积Rail_dvolDemSysNom' '' } %GIDa_73831af3_0478_4c8d_b3f3_fdf3f80fb0df  Port=5
  wires:
  Constant2/1 -> Divide1/2
  Add3/1 -> Rail_dvolDemSysNom/1
  Rail_dvolDemInjNom/1 -> Add3/2
  Add2/1 -> Rail_dvolDemSysMax/1
  Rail_dvolDemInjMax/1 -> Add2/2
  Constant1/1 -> Divide3/2
  EngDa_tiEngOn_mp/1 -> Divide3/1
  Divide3/1 -> Rail_facLeakEngOn_CUR/1  "Rail_tiLeakEngOn_mp"
  Add1/1 -> Rail_dvolLeakSumMax/1, Add2/1
  Divide2/1 -> Add1/2
  Rail_facLeakEngOn_CUR/1 -> Divide2/2  "Rail_facLeakAged_mp"
  Add6/1 -> Rail_dvolLeakSum/1
  Constant3/1 -> Add6/2, Add1/1
  Divide1/1 -> Rail_dvolLeak/1, Add6/1, Divide2/1, Add3/1  "Rail_dvolLeak"
  Divide5/1 -> Divide1/1  "Rail_dvolLeakCyl_mp"
  Rail_facLeakTempCor_CUR/1 -> Divide5/2  "Rail_facLeakTempCor_mp"
  Rail_dvolLeak_CUR/1 -> Divide5/1
  FuelT_tFlSys/1 -> Rail_facLeakTempCor_CUR/1
  Rail_pSetPoint/1 -> Delay1/1
  Delay1/1 -> Rail_dvolLeak_CUR/1

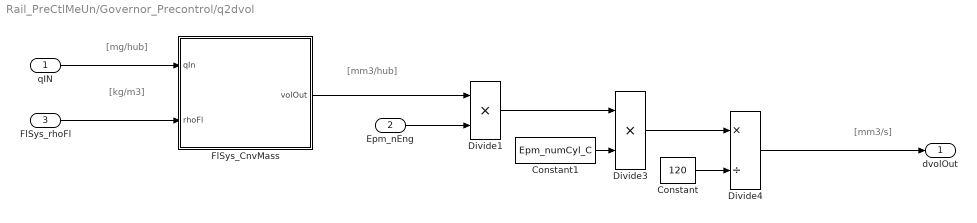
== system Rail_PreCtlMeUn/Governor_Precontrol/q2dvol ==
  note: [mg/hub]
  note: [kg/m3]
  note: [mm3/hub]
  note: [mm3/s]
  qIN : Inport
  Epm_nEng : Inport  Port=2
  FlSys_rhoFl : Inport  Port=3
  Constant : Constant  Value=120  OutDataTypeStr=uint16
  Constant1 : Constant  Value=Epm_numCyl_C
  Divide1 : Product  Inputs=**  OutDataTypeStr=fixdt(1,32,5)  SaturateOnIntegerOverflow=on
  Divide3 : Product  Inputs=**  OutDataTypeStr=fixdt(1,32,5)  SaturateOnIntegerOverflow=on
  Divide4 : Product  Inputs=*/  OutDataTypeStr=Inherit: Inherit via back propagation  SaturateOnIntegerOverflow=on
  FlSys_CnvMass : Subsystem
  dvolOut : Outport
  wires:
  Divide3/1 -> Divide4/1
  Divide1/1 -> Divide3/1
  Constant1/1 -> Divide3/2
  Epm_nEng/1 -> Divide1/2
  Constant/1 -> Divide4/2
  FlSys_CnvMass/1(volOut) -> Divide1/1
  Divide4/1 -> dvolOut/1
  qIN/1 -> FlSys_CnvMass/1(qIn)
  FlSys_rhoFl/1 -> FlSys_CnvMass/2(rhoFl)

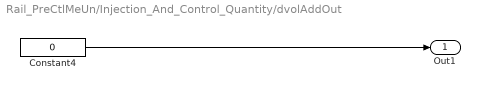
== system Rail_PreCtlMeUn/Injection_And_Control_Quantity/dvolAddOut ==
  Constant4 : Constant  Value=0  OutDataTypeStr=FuelVol_mm3_s
  Out1 : Outport
  wires:
  Constant4/1 -> Out1/1

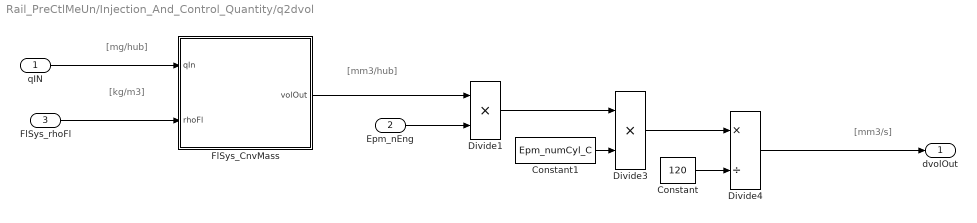
== system Rail_PreCtlMeUn/Injection_And_Control_Quantity/q2dvol ==
  note: [mg/hub]
  note: [kg/m3]
  note: [mm3/hub]
  note: [mm3/s]
  qIN : Inport
  Epm_nEng : Inport  Port=2
  FlSys_rhoFl : Inport  Port=3
  Constant : Constant  Value=120  OutDataTypeStr=uint16
  Constant1 : Constant  Value=Epm_numCyl_C
  Divide1 : Product  Inputs=**  OutDataTypeStr=fixdt(1,32,5)  SaturateOnIntegerOverflow=on
  Divide3 : Product  Inputs=**  OutDataTypeStr=fixdt(1,32,5)  SaturateOnIntegerOverflow=on
  Divide4 : Product  Inputs=*/  OutDataTypeStr=Inherit: Inherit via back propagation  SaturateOnIntegerOverflow=on
  FlSys_CnvMass : Subsystem
  dvolOut : Outport
  wires:
  Divide3/1 -> Divide4/1
  Divide1/1 -> Divide3/1
  Constant1/1 -> Divide3/2
  Epm_nEng/1 -> Divide1/2
  Constant/1 -> Divide4/2
  FlSys_CnvMass/1(volOut) -> Divide1/1
  Divide4/1 -> dvolOut/1
  qIN/1 -> FlSys_CnvMass/1(qIn)
  FlSys_rhoFl/1 -> FlSys_CnvMass/2(rhoFl)

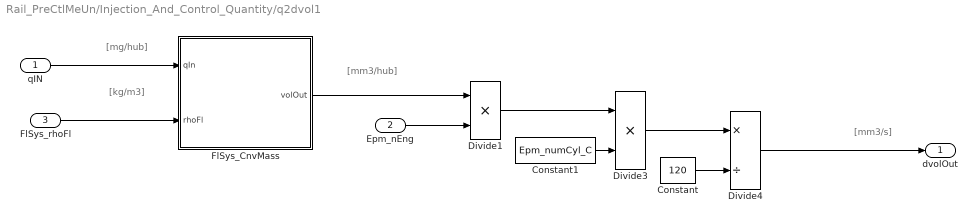
== system Rail_PreCtlMeUn/Injection_And_Control_Quantity/q2dvol1 ==
  note: [mm3/s]
  note: [mm3/hub]
  note: [kg/m3]
  note: [mg/hub]
  qIN : Inport
  Epm_nEng : Inport  Port=2
  FlSys_rhoFl : Inport  Port=3
  Constant : Constant  Value=120  OutDataTypeStr=uint16
  Constant1 : Constant  Value=Epm_numCyl_C
  Divide1 : Product  Inputs=**  OutDataTypeStr=fixdt(1,32,5)  SaturateOnIntegerOverflow=on
  Divide3 : Product  Inputs=**  OutDataTypeStr=fixdt(1,32,5)  SaturateOnIntegerOverflow=on
  Divide4 : Product  Inputs=*/  OutDataTypeStr=Inherit: Inherit via back propagation  SaturateOnIntegerOverflow=on
  FlSys_CnvMass : Subsystem
  dvolOut : Outport
  wires:
  FlSys_rhoFl/1 -> FlSys_CnvMass/2(rhoFl)
  qIN/1 -> FlSys_CnvMass/1(qIn)
  Divide4/1 -> dvolOut/1
  FlSys_CnvMass/1(volOut) -> Divide1/1
  Constant/1 -> Divide4/2
  Epm_nEng/1 -> Divide1/2
  Constant1/1 -> Divide3/2
  Divide1/1 -> Divide3/1
  Divide3/1 -> Divide4/1

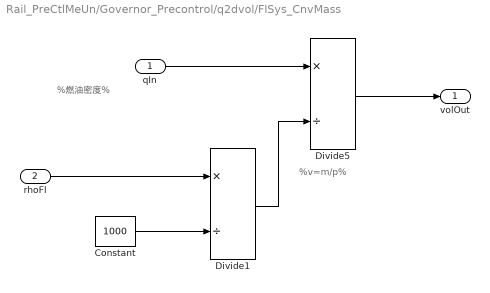
== system Rail_PreCtlMeUn/Governor_Precontrol/q2dvol/FlSys_CnvMass ==
  note: %燃油密度%
  note: %v=m/p%
  qIn : Inport
  rhoFl : Inport  Port=2
  Constant : Constant  Value=1000  OutDataTypeStr=uint16
  Divide1 : Product  Inputs=*/  OutDataTypeStr=fixdt(1,16,7)  SaturateOnIntegerOverflow=on
  Divide5 : Product  Inputs=*/  OutDataTypeStr=FuelMass_mm3_hub  SaturateOnIntegerOverflow=on
  volOut : Outport
  wires:
  Divide1/1 -> Divide5/2
  Constant/1 -> Divide1/2
  qIn/1 -> Divide5/1
  rhoFl/1 -> Divide1/1
  Divide5/1 -> volOut/1

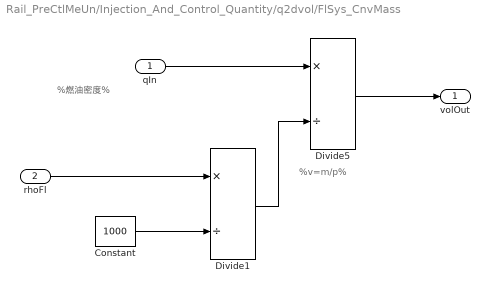
== system Rail_PreCtlMeUn/Injection_And_Control_Quantity/q2dvol/FlSys_CnvMass ==
  note: %燃油密度%
  note: %v=m/p%
  qIn : Inport
  rhoFl : Inport  Port=2
  Constant : Constant  Value=1000  OutDataTypeStr=uint16
  Divide1 : Product  Inputs=*/  OutDataTypeStr=fixdt(1,16,7)  SaturateOnIntegerOverflow=on
  Divide5 : Product  Inputs=*/  OutDataTypeStr=FuelMass_mm3_hub  SaturateOnIntegerOverflow=on
  volOut : Outport
  wires:
  Divide1/1 -> Divide5/2
  Constant/1 -> Divide1/2
  qIn/1 -> Divide5/1
  rhoFl/1 -> Divide1/1
  Divide5/1 -> volOut/1

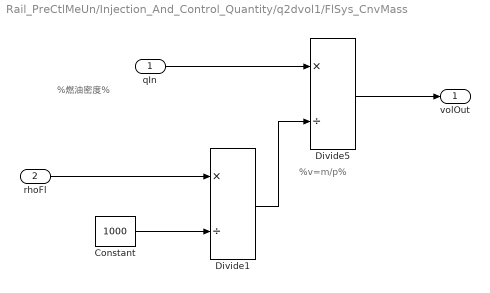
== system Rail_PreCtlMeUn/Injection_And_Control_Quantity/q2dvol1/FlSys_CnvMass ==
  note: %v=m/p%
  note: %燃油密度%
  qIn : Inport
  rhoFl : Inport  Port=2
  Constant : Constant  Value=1000  OutDataTypeStr=uint16
  Divide1 : Product  Inputs=*/  OutDataTypeStr=fixdt(1,16,7)  SaturateOnIntegerOverflow=on
  Divide5 : Product  Inputs=*/  OutDataTypeStr=FuelMass_mm3_hub  SaturateOnIntegerOverflow=on
  volOut : Outport
  wires:
  Divide5/1 -> volOut/1
  rhoFl/1 -> Divide1/1
  qIn/1 -> Divide5/1
  Constant/1 -> Divide1/2
  Divide1/1 -> Divide5/2
